simulink model "Impresora_2inputs_7"  (R2022a)
settings: Solver=VariableStepAuto  StartTime=0.0  StopTime=50  RelTol=1e-3
libraries: fuzblock x1
settings Model: Creator=DiegoPaez  LastModifiedBy=SEBASTIANDIAZPABON
settings SolverCC: ZeroCrossAlgorithm=Adaptive  AlgebraicLoopSolver=TrustRegion
settings DataIOCC: ReturnWorkspaceOutputs=off
settings DebuggingCC: IgnoredZcDiagnostic=none  UnconnectedInputMsg=warning  UnconnectedOutputMsg=warning  UnconnectedLineMsg=warning  SFMachineParentedDataDiag=warning
settings RTWCC: DLArmComputeVersion=19.05

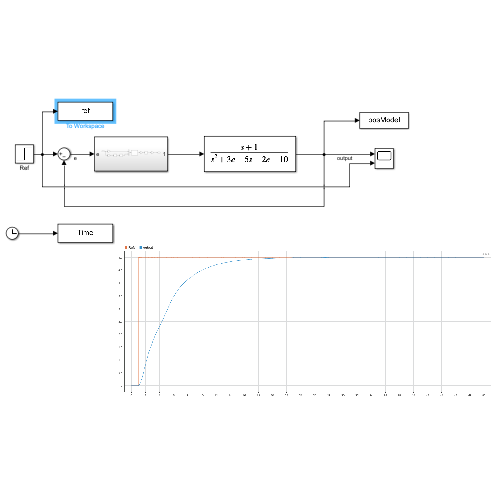
[thumbnail: Simulink's stored preview of the top-level diagram]
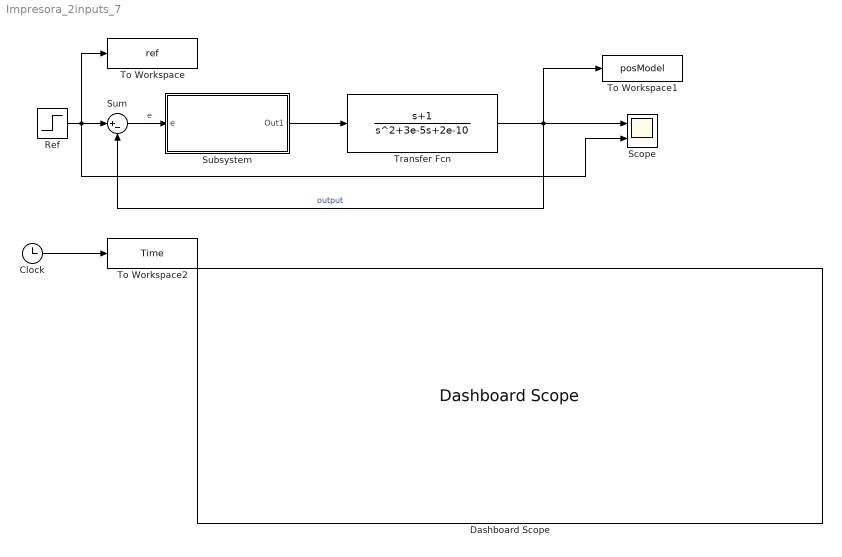
== system Impresora_2inputs_7 ==
  Clock : Clock
  Dashboard Scope : DashboardScope  Ymin=0  Ymax=7
  Ref : Step  After=5  SampleTime=0
  Scope : Scope  NumInputPorts=2
  Subsystem : Subsystem
  Sum : Sum  Inputs=|+-
  To Workspace : ToWorkspace  VariableName=ref  SampleTime=1
      settings: Save2DSignal=2-D array (concatenate along first dimension)
  To Workspace1 : ToWorkspace  VariableName=posModel  SampleTime=1
      settings: Save2DSignal=2-D array (concatenate along first dimension)
  To Workspace2 : ToWorkspace  VariableName=Time  SampleTime=1
      settings: Save2DSignal=2-D array (concatenate along first dimension)
  Transfer Fcn : TransferFcn  Numerator=[1 1]  Denominator=[1 3e-5 2e-10]
  wires:
  Ref/1 -> Scope/2, Sum/1, To Workspace/1
  Transfer Fcn/1 -> Sum/2, Scope/1, To Workspace1/1  "output"
  Clock/1 -> To Workspace2/1
  Sum/1 -> Subsystem/1(e)  "e"
  Subsystem/1(Out1) -> Transfer Fcn/1

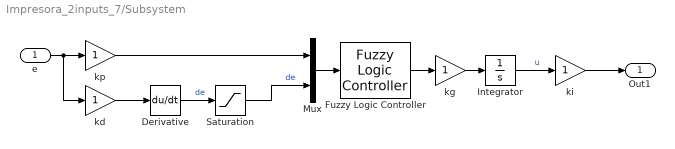
== system Impresora_2inputs_7/Subsystem ==
  e : Inport
  Derivative : Derivative
  Fuzzy Logic Controller : fuzblock/Fuzzy Logic  Controller  FIS='Impresora_2inputs.fis'  OutputSampleNumber=101  DataType=double  FuzzifiedInputs=off  RuleFiringStrengths=off  RuleOutputs=off  AggregatedOutputs=off  SimulateUsing=Interpreted execution  OutOfRangeInputValueMessage=warning  NoRuleFiredMessage=warning  EmptyOutputFuzzySetMessage=warning
  Integrator : Integrator
  Mux : Mux  Inputs=2
  Saturation : Saturate  UpperLimit=3.9  LowerLimit=-3.9
  kd : Gain
  kg : Gain
  ki : Gain
  kp : Gain
  Out1 : Outport
  wires:
  kd/1 -> Derivative/1
  kg/1 -> Integrator/1
  Derivative/1 -> Saturation/1  "de"
  e/1 -> kp/1, kd/1
  ki/1 -> Out1/1
  Saturation/1 -> Mux/2  "de"
  Mux/1 -> Fuzzy Logic Controller/1
  Fuzzy Logic Controller/1 -> kg/1
  kp/1 -> Mux/1
  Integrator/1 -> ki/1  "u"
